simulink model "sim11ex3"  (Simulink 4.00)
settings: Solver=ode45  SolverMode=SingleTasking  StartTime=0.0  StopTime=3  MaxStep=.0250  RelTol=1e-3  AbsTol=1e-3
settings Model: LastModifiedBy=saadat  SaveTime=off  SaveOutput=off  LimitDataPoints=off  RTWTemplateMakefile=grt_vc.tmf  ExtModeTrigMode=oneshot  ExtModeArmWhenConnect=off

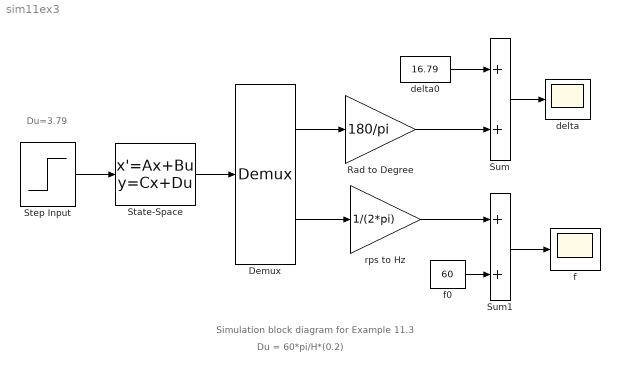
== system sim11ex3 ==
  note: Du=3.79
  note: Du = 60*pi/H*(0.2)
  note: Simulation block diagram for Example 11.3
  Demux : Demux  Outputs=2  BusSelectionMode=off
  "Rad to Degree  " : Gain  Gain=180/pi  Multiplication=Element-wise(K.*u)  SaturateOnIntegerOverflow=on
  State-Space : StateSpace  A="[0    1;  -37.7061   -2.6169 ]"  B="[0;   1]"  C=eye(2)  D=zeros(2, 1)  X0=0  AbsoluteTolerance=auto  Realization=auto
  Step Input : Step  Time=0  Before=0  After=pi*60/9.84*.2  SampleTime=0
  Sum : Sum  Inputs=++  SaturateOnIntegerOverflow=on
  Sum1 : Sum  Inputs=++  SaturateOnIntegerOverflow=on
  delta : Scope
      settings: TickLabels=on  TimeRange=3  YMin=16  YMax=26  SaveToWorkspace=off  SaveName=ScopeData  DataFormat=Array  LimitDataPoints=on  MaxDataPoints=5000
  delta0 : Constant  Value=16.79
  f : Scope
      settings: TickLabels=on  TimeRange=3  YMin=59.96  YMax=60.08  SaveToWorkspace=off  SaveName=ScopeData  DataFormat=Array  LimitDataPoints=on  MaxDataPoints=5000
  f0 : Constant  Value=60
  rps to Hz : Gain  Gain=1/(2*pi)  Multiplication=Element-wise(K.*u)  SaturateOnIntegerOverflow=on
  wires:
  f0/1 -> Sum1/2
  rps to Hz/1 -> Sum1/1
  delta0/1 -> Sum/1
  Demux/2 -> rps to Hz/1
  Sum/1 -> delta/1
  "Rad to Degree  "/1 -> Sum/2
  Demux/1 -> "Rad to Degree  "/1
  Sum1/1 -> f/1
  State-Space/1 -> Demux/1
  Step Input/1 -> State-Space/1
